simulink model "chap1_3"  (R2012b)
settings: Solver=ode45  StartTime=0.0  StopTime=10.0  RelTol=1e-3
settings Model: Creator=Administrator  LastModifiedBy=Administrator

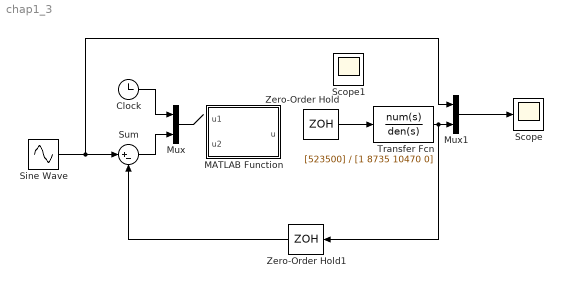
== system chap1_3 ==
  Clock : Clock
  MATLAB Function : MATLAB Function  TreatAsAtomicUnit=on
  Mux : Mux  Inputs=2
  Mux1 : Mux  Inputs=2
  Scope : Scope
  Scope1 : Scope
  Sine Wave : Sin  SampleTime=0.001
  Sum : Sum  Inputs=|+-
  Transfer Fcn : TransferFcn  Numerator=[523500]  Denominator=[1 8735 10470 0]
  Zero-Order Hold : ZeroOrderHold
  Zero-Order Hold1 : ZeroOrderHold
  wires:
  Clock/1 -> Mux/1
  Sum/1 -> Mux/2
  Sine Wave/1 -> Mux1/1, Sum/1
  Mux/1 -> ?
  Transfer Fcn/1 -> Zero-Order Hold1/1, Mux1/2
  Mux1/1 -> Scope/1
  ? -> Scope1/1, Zero-Order Hold/1
  Zero-Order Hold/1 -> Transfer Fcn/1
  Zero-Order Hold1/1 -> Sum/2

== matlab function chap1_3/MATLAB Function ==
  data: u output; u1 input; u2 input
function u  = pidsimf(u1,u2)
%#codegen
persistent pidmat errori error_1
if u1==0
    errori=0;
    error_l=0;
end
ts=0.001;
kp=1.5;
ki=2.0;
kd=0.05;

error=u2;
errori=errori+error*ts;
errord=(error-error_l)/ts;

u=kp*error+ki*errori+kd*errord;
error_l=error;
